simulink model "ctsdm_3stage_fir_firc"  (R2021a)
settings: Solver=VariableStepAuto  StartTime=0.0  StopTime=time  RelTol=1e-3
undefined symbols (not defined in the file or in its folder): c1, c2, c3, fin, fs, k1, k2, k3, Mpoints, osr, Ts, xc
libraries: SDtoolbox x1
settings Model: Creator=weihaoyu  LastModifiedBy=weihaoyu

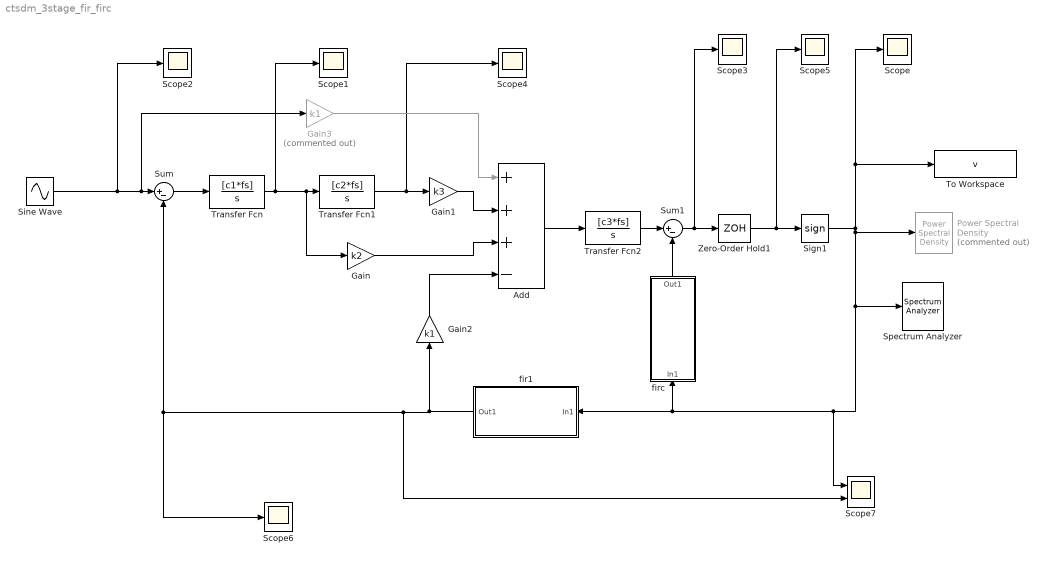
== system ctsdm_3stage_fir_firc ==
  Add : Sum  Inputs=+++-
  Gain : Gain  Gain=k2
  Gain1 : Gain  Gain=k3
  Gain2 : Gain  Gain=k1
  Gain3 : Gain  Commented=on  Gain=k1
  Power Spectral Density : SDtoolbox/Power Spectral Density  Commented=on  SN=2  Fs=fs  fBL=0  fBH=fs/(2*osr)  Fin=fin  N=Mpoints  Ntransient=10  VW=off  savename=savemat  Scale_type=logarithmic
  Scope{,1..6} (7 alike) : Scope
  Scope7 : Scope  NumInputPorts=2
  Sign1 : Signum
  Sine Wave : Sin  Amplitude=0.8  Frequency=fin*2*pi  SampleTime=0
  Spectrum Analyzer : SpectrumAnalyzer
  Sum : Sum  Inputs=|+-
  Sum1 : Sum  Inputs=|+-
  To Workspace : ToWorkspace  VariableName=v  SampleTime=1/fs
  Transfer Fcn : TransferFcn  Numerator=[c1*fs]  Denominator=[1 0]
  Transfer Fcn1 : TransferFcn  Numerator=[c2*fs]  Denominator=[1 0]
  Transfer Fcn2 : TransferFcn  Numerator=[c3*fs]  Denominator=[1 0]
  Zero-Order Hold1 : ZeroOrderHold  SampleTime=1/fs
  fir1 : Subsystem
  firc : Subsystem
  wires:
  Transfer Fcn/1 -> Scope1/1, Gain/1, Transfer Fcn1/1
  Transfer Fcn1/1 -> Gain1/1, Scope4/1
  Gain1/1 -> Add/2
  Gain/1 -> Add/3
  Add/1 -> Transfer Fcn2/1
  Gain2/1 -> Add/4
  Sine Wave/1 -> Scope2/1, Gain3/1, Sum/1
  Sum/1 -> Transfer Fcn/1
  Gain3/1 -> Add/1
  Zero-Order Hold1/1 -> Sign1/1, Scope5/1
  Transfer Fcn2/1 -> Sum1/1
  Sum1/1 -> Scope3/1, Zero-Order Hold1/1
  firc/1(Out1) -> Sum1/2
  fir1/1(Out1) -> Scope7/2, Sum/2, Scope6/1, Gain2/1
  Sign1/1 -> Power Spectral Density/1, Scope7/1, fir1/1(In1), firc/1(In1), Spectrum Analyzer/1, To Workspace/1, Scope/1

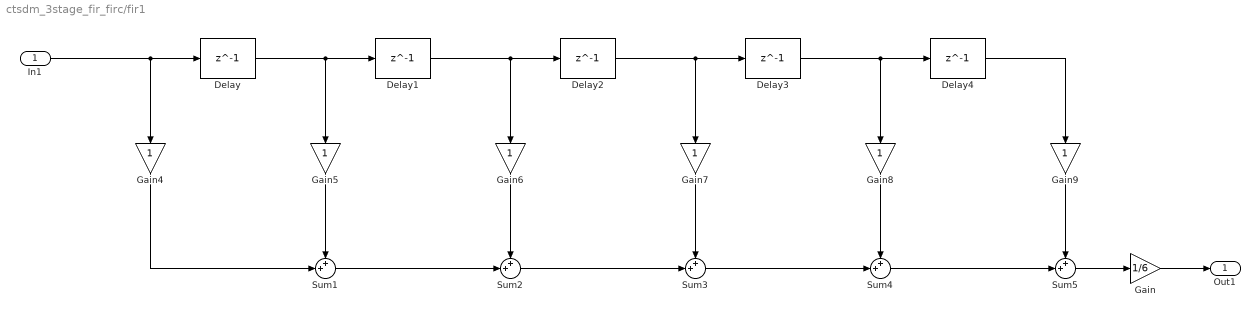
== system ctsdm_3stage_fir_firc/fir1 ==
  In1 : Inport
  Delay{,1..4} (5 alike) : Delay  DelayLength=1  InputProcessing=Columns as channels (frame based)  SampleTime=Ts
  Gain : Gain  Gain=1/6
  Gain{4..9} (6 alike) : Gain
  Sum{1..5} (5 alike) : Sum  Inputs=++|
  Out1 : Outport
  wires:
  Gain/1 -> Out1/1
  Gain9/1 -> Sum5/1
  Sum5/1 -> Gain/1
  Gain6/1 -> Sum2/1
  Sum4/1 -> Sum5/2
  Sum2/1 -> Sum3/2
  Sum1/1 -> Sum2/2
  Gain4/1 -> Sum1/2
  Gain5/1 -> Sum1/1
  In1/1 -> Delay/1, Gain4/1
  Gain8/1 -> Sum4/1
  Delay2/1 -> Delay3/1, Gain7/1
  Delay3/1 -> Delay4/1, Gain8/1
  Gain7/1 -> Sum3/1
  Sum3/1 -> Sum4/2
  Delay1/1 -> Delay2/1, Gain6/1
  Delay4/1 -> Gain9/1
  Delay/1 -> Gain5/1, Delay1/1

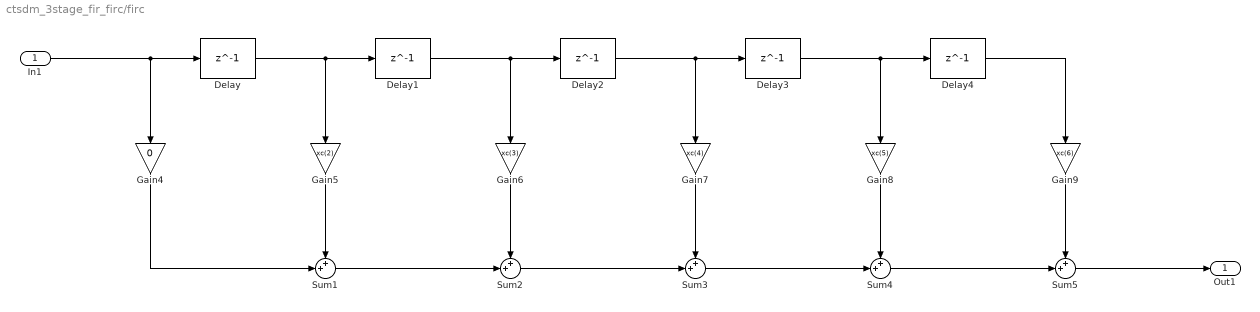
== system ctsdm_3stage_fir_firc/firc ==
  In1 : Inport
  Delay{,1..4} (5 alike) : Delay  DelayLength=1  InputProcessing=Columns as channels (frame based)  SampleTime=Ts
  Gain4 : Gain  Gain=0
  Gain5 : Gain  Gain=xc(2)
  Gain6 : Gain  Gain=xc(3)
  Gain7 : Gain  Gain=xc(4)
  Gain8 : Gain  Gain=xc(5)
  Gain9 : Gain  Gain=xc(6)
  Sum{1..5} (5 alike) : Sum  Inputs=++|
  Out1 : Outport
  wires:
  Gain9/1 -> Sum5/1
  Sum5/1 -> Out1/1
  Gain6/1 -> Sum2/1
  Sum4/1 -> Sum5/2
  Sum2/1 -> Sum3/2
  Sum1/1 -> Sum2/2
  Gain4/1 -> Sum1/2
  Gain5/1 -> Sum1/1
  In1/1 -> Delay/1, Gain4/1
  Gain8/1 -> Sum4/1
  Delay2/1 -> Delay3/1, Gain7/1
  Delay3/1 -> Delay4/1, Gain8/1
  Gain7/1 -> Sum3/1
  Sum3/1 -> Sum4/2
  Delay1/1 -> Delay2/1, Gain6/1
  Delay4/1 -> Gain9/1
  Delay/1 -> Gain5/1, Delay1/1
